simulink model "GPCA_Logging"  (Simulink 8.7)
settings: Solver=VariableStepAuto  StartTime=0.0  StopTime=10.0  RelTol=1e-3
libraries: simulink x2
settings Model: Creator=bourbouh  LastModifiedBy=bourbouh
settings DataIOCC: LimitDataPoints=off  SaveFormat=Dataset
settings DebuggingCC: UnderspecifiedInitializationDetection=Simplified  MergeDetectMultiDrivingBlocksExec=error
settings HardwareCC: ProdBitPerPointer=64  ProdLargestAtomicFloat=Float  ProdIntDivRoundTo=Zero  ProdEndianess=LittleEndian  ProdWordSize=64  ProdHWDeviceType=Intel->x86-64 (Windows64)
settings ModelReferenceCC: PropagateSignalLabelsOutOfModel=on
settings ConfigComp: CovModelRefEnable=off

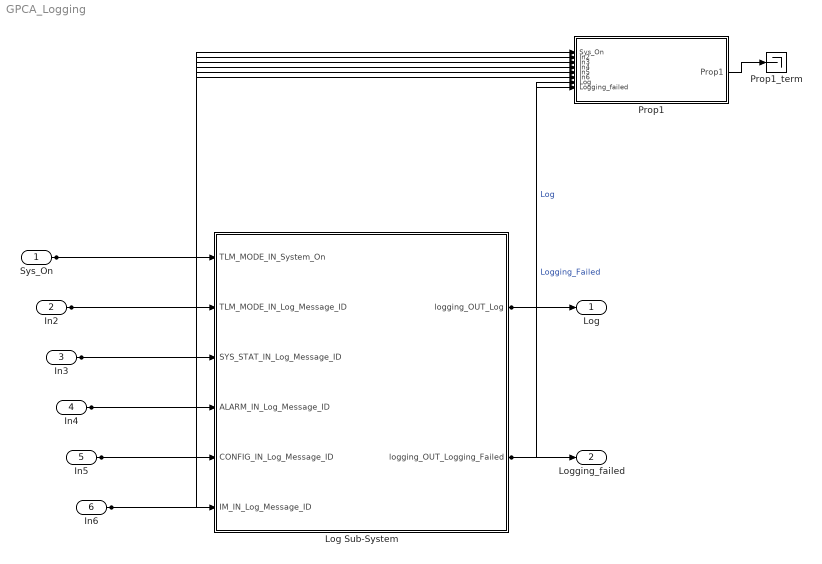
== system GPCA_Logging ==
  Sys_On : Inport
  In2 : Inport  Port=2
  In3 : Inport  Port=3
  In4 : Inport  Port=4
  In5 : Inport  Port=5
  In6 : Inport  Port=6
  Log Sub-System : Stateflow chart  TreatAsAtomicUnit=on
  Prop1 : Subsystem  TreatAsAtomicUnit=on  mask(Observer){AnnotationType=ensures, ObserverType=[]}
      mask prompts: AnnotationType "Type of annotation (pre/post...)"; ObserverType "Observer type"
      mask help:
      | Set an observer for the system.
      | The annotation type parameter sets the type of observer:
      | - requires : pre-condition
      | - ensures : post-condition
      | - assert : an assertion
      | - observer : the observer computes a special type of properties
      mask TypeOptions AnnotationType: ensures | requires | assert | observer
      mask Callback AnnotationType:
      | paramStr = get_param(gcb, 'MaskValues');
      | if strcmp(paramStr{1}(1),'o')
      | set_param(gcb,'MaskVisibilities',{'on';'on'});
      | paramStr{2} = 'ellipsoid';
      | set_param(gcb,'MaskValues',paramStr);
      | else
      | set_param(gcb,'MaskVisibilities',{'on';'off'});
      | end
      | clear paramStr;
      mask Callback ObserverType:
      | paramStr = get_param(gcb, 'MaskValues');
      | if strcmp(paramStr{1}(1),'o')
      | set_param(gcb,'MaskVisibilities',{'on';'on'});
      | paramStr{2} = 'ellipsoid';
      | set_param(gcb,'MaskValues',paramStr);
      | else
      | set_param(gcb,'MaskVisibilities',{'on';'off'});
      | end
      | clear paramStr;
      mask Display:
      | color('black')
      | text(0.5, 0.5, ['Property: ''' get_param(gcb,'name') ''''], 'horizontalAlignment', 'center');
      | text(0.99, 0.03, '{\bf\fontsize{12}SAFE}', 'hor', 'right', 'ver', 'bottom', 'texmode', 'on');
  Prop1_term : Terminator
  Log : Outport
  Logging_failed : Outport  Port=2
  wires:
  Sys_On/1 -> Log Sub-System/1(TLM_MODE_IN_System_On), Prop1/1(Sys_On)
  In2/1 -> Log Sub-System/2(TLM_MODE_IN_Log_Message_ID), Prop1/2(In2)
  In3/1 -> Log Sub-System/3(SYS_STAT_IN_Log_Message_ID), Prop1/3(In3)
  In4/1 -> Log Sub-System/4(ALARM_IN_Log_Message_ID), Prop1/4(In4)
  In5/1 -> Log Sub-System/5(CONFIG_IN_Log_Message_ID), Prop1/5(In5)
  In6/1 -> Log Sub-System/6(IM_IN_Log_Message_ID), Prop1/6(In6)
  Log Sub-System/1(logging_OUT_Log) -> Log/1, Prop1/7(Log)  "Log"
  Log Sub-System/2(logging_OUT_Logging_Failed) -> Logging_failed/1, Prop1/8(Logging_failed)  "Logging_Failed"
  Prop1/1(Prop1) -> Prop1_term/1

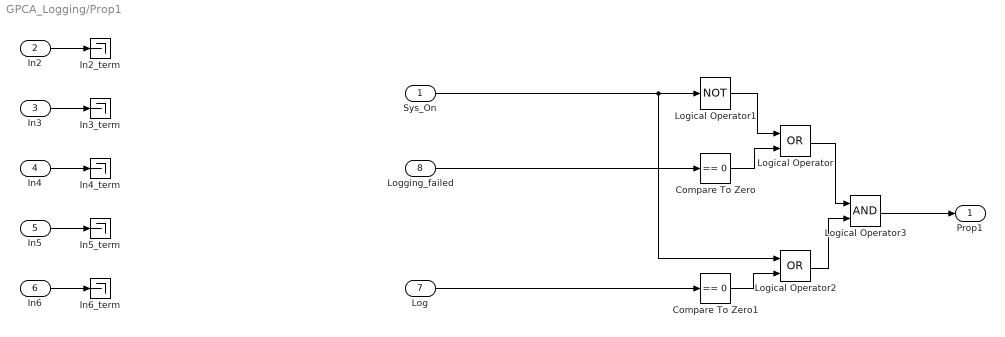
== system GPCA_Logging/Prop1 ==
  Sys_On : Inport
  In2 : Inport  Port=2
  In3 : Inport  Port=3
  In4 : Inport  Port=4
  In5 : Inport  Port=5
  In6 : Inport  Port=6
  Log : Inport  Port=7
  Logging_failed : Inport  Port=8
  Compare To Zero : simulink/Logic and Bit Operations/Compare To Zero  relop===  OutDataTypeStr=boolean
  Compare To Zero1 : simulink/Logic and Bit Operations/Compare To Zero  relop===  OutDataTypeStr=boolean
  In2_term : Terminator
  In3_term : Terminator
  In4_term : Terminator
  In5_term : Terminator
  In6_term : Terminator
  Logical Operator : Logic  Operator=OR  AllPortsSameDT=off  OutDataTypeStr=boolean
  Logical Operator1 : Logic  Operator=NOT  AllPortsSameDT=off  OutDataTypeStr=boolean
  Logical Operator2 : Logic  Operator=OR  AllPortsSameDT=off  OutDataTypeStr=boolean
  Logical Operator3 : Logic  AllPortsSameDT=off  OutDataTypeStr=boolean
  Prop1 : Outport
  wires:
  Sys_On/1 -> Logical Operator2/1, Logical Operator1/1
  In2/1 -> In2_term/1
  In3/1 -> In3_term/1
  In4/1 -> In4_term/1
  In5/1 -> In5_term/1
  In6/1 -> In6_term/1
  Log/1 -> Compare To Zero1/1
  Logging_failed/1 -> Compare To Zero/1
  Logical Operator/1 -> Logical Operator3/1
  Logical Operator1/1 -> Logical Operator/1
  Compare To Zero/1 -> Logical Operator/2
  Compare To Zero1/1 -> Logical Operator2/2
  Logical Operator2/1 -> Logical Operator3/2
  Logical Operator3/1 -> Prop1/1

== stateflow chart Log Sub-System ==
  state NOT_ON
    entry: logging_OUT_Log=0;
    during : logging_OUT_Log=0;
    exit: logging_OUT_Log=0;
  state LOG
    entry: logging_OUT_Logging_Failed=0;
    logging_OUT_Log= writeLog(TLM_MODE_IN_Log_Message_ID, SYS_STAT_IN_Log_Message_ID, ALARM_IN_Log_Message_ID, CONFIG_IN_Log_Message_ID, IM_IN_Log_Message_ID)
    during: logging_OUT_Logging_Failed=0;
    logging_OUT_Log= writeLog(TLM_MODE_IN_Log_Message_ID, SYS_STAT_IN_Log_Message_ID, ALARM_IN_Log_Message_ID, CONFIG_IN_Log_Message_ID, IM_IN_Log_Message_ID)
    exit: logging_OUT_Logging_Failed=0;
    logging_OUT_Log= writeLog(TLM_MODE_IN_Log_Message_ID, SYS_STAT_IN_Log_Message_ID, ALARM_IN_Log_Message_ID, CONFIG_IN_Log_Message_ID, IM_IN_Log_Message_ID)
  note: Functionality shall be added later. For now its just a place holder
  state logging_OUT_Log= writeLog(TLM_MODE_IN_Log_Message_ID, SYS_STAT_IN_Log_Message_ID, ALARM_IN_Log_Message_ID, CONFIG_IN_Log_Message_ID, IM_IN_Log_Message_ID) [function]
    (default) -> (junction 13) : {logging_OUT_Log=0;}
    (junction 13) -> (junction 14) : [(TLM_MODE_IN_Log_Message_ID > 0) || (SYS_STAT_IN_Log_Message_ID > 0)  || (ALARM_IN_Log_Message_ID > 0)  ||  (CONFIG_IN_Log_Message_ID > 0)  || (IM_IN_Log_Message_ID > 0)]{logging_OUT_Log=1;}
  (default) -> NOT_ON [order 2]
  (default) -> LOG [order 1] : [TLM_MODE_IN_System_On]
  NOT_ON -> LOG : [TLM_MODE_IN_System_On]
  LOG -> NOT_ON : [!TLM_MODE_IN_System_On]
  data: logging_OUT_Log function_output uint8; TLM_MODE_IN_Log_Message_ID function_input uint8; SYS_STAT_IN_Log_Message_ID function_input uint8; ALARM_IN_Log_Message_ID function_input uint8; CONFIG_IN_Log_Message_ID function_input uint8; IM_IN_Log_Message_ID function_input uint8; TLM_MODE_IN_System_On input boolean; TLM_MODE_IN_Log_Message_ID input uint8; SYS_STAT_IN_Log_Message_ID input uint8; ALARM_IN_Log_Message_ID input uint8; CONFIG_IN_Log_Message_ID input uint8; logging_OUT_Log output uint8; logging_OUT_Logging_Failed output boolean; IM_IN_Log_Message_ID input uint8
